simulink model "Timer"  (R2021a)
settings: Solver=ode3  StartTime=0.0  StopTime=10.0  FixedStep=0.01  RelTol=1e-3
settings Model: Creator=Oceaner  LastModifiedBy=Oceaner

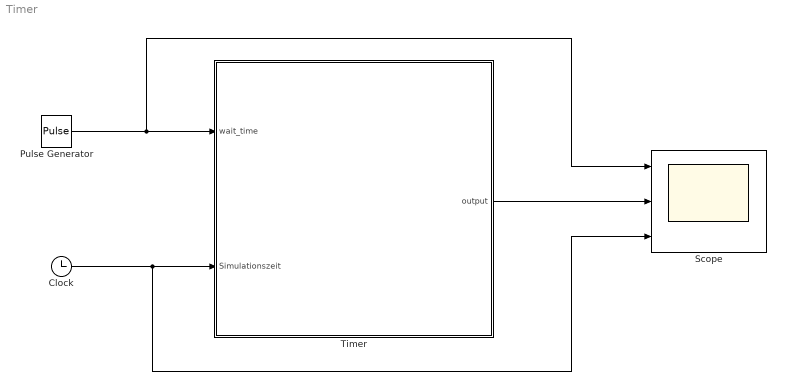
== system Timer ==
  Clock : Clock
  Pulse Generator : DiscretePulseGenerator  PulseType=Time based  Period=3  PulseWidth=50
  Scope : Scope  NumInputPorts=3
  Timer : Stateflow chart  TreatAsAtomicUnit=on
  wires:
  Pulse Generator/1 -> Scope/1, Timer/1(wait_time)
  Clock/1 -> Scope/3, Timer/2(Simulationszeit)
  Timer/1(output) -> Scope/2

== stateflow chart Timer/Timer ==
  state b
    en:output=1;
  state warte
  state a
    en:output=0;
  (default) -> a
  warte -> b : after(1,sec)
  a -> warte : [wait_time==1]
  b -> a
  data: wait_time input; Simulationszeit input; output output
